simulink model "verify_THB_P_adapter_mdl"  (R2016b)
settings: Solver=ode45  StartTime=0  StopTime=600  MaxStep=10  RelTol=1e-3  EnableMultiTasking=on
libraries: carnot x2, simulink x1
settings Model: Creator=drhf  LastModifiedBy=drhf
settings DataIOCC: SaveFormat=Array  SignalLoggingSaveFormat=ModelDataLogs
settings OptimizationCC: ExpressionDepthLimit=2147483647  LifeSpan=inf
settings DebuggingCC: UnderspecifiedInitializationDetection=Classic  MergeDetectMultiDrivingBlocksExec=none  SolverPrmCheckMsg=warning  FcnCallInpInsideContextMsg=warning  StateNameClashWarn=warning  SFUnexpectedBacktrackingDiag=warning  SFNoUnconditionalDefaultTransitionDiag=warning  SFExecutionAtInitializationDiag=none
settings HardwareCC: ProdBitPerPointer=32  ProdBitPerSizeT=32  ProdBitPerPtrDiffT=32  ProdLargestAtomicFloat=None  ProdIntDivRoundTo=Undefined  ProdEndianess=Unspecified  ProdWordSize=32  ProdHWDeviceType=32-bit Generic
settings ModelReferenceCC: PropagateSignalLabelsOutOfModel=off
settings GRTTargetCC: TargetLangStandard=C89/C90 (ANSI)  GeneratePreprocessorConditionals=Disable all  CombineOutputUpdateFcns=off  GRTInterface=on
settings ConfigComp: CovMetricSettings=dw  CovHtmlReporting=on  CovSaveCumulativeToWorkspaceVar=on  CovSaveSingleToWorkspaceVar=on  CovExternalEMLEnable=off

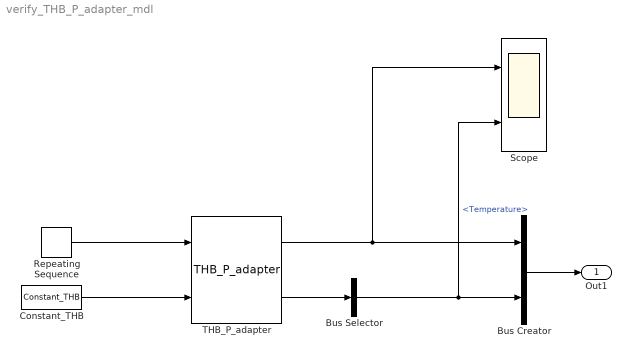
== system verify_THB_P_adapter_mdl ==
  Bus Creator : BusCreator  Inputs=2
  Bus Selector : BusSelector  OutputSignals=Temperature
  Constant_THB : carnot/Source/Simple/Constant_THB  t=40  mdot=600/3600  p=1e5  mID=No Pressure Drop  fluid=Water  mix=0  mix2=0  mix3=0  dia=0.02  hgt=0
  Repeating Sequence : simulink/Sources/Repeating Sequence  rep_seq_t=[0 100 200 400 500 600]  rep_seq_y=[20 20 30 30 10 10]
  Scope : Scope  NumInputPorts=2
  THB_P_adapter : carnot/Load/Houses/ventilation_heating/THB_P_adapter  mass=1  ua=800*5*5/0.2*0.022*3.1415  t0=20
  Out1 : Outport
  wires:
  THB_P_adapter/2 -> Bus Selector/1
  Constant_THB/1 -> THB_P_adapter/2
  Repeating Sequence/1 -> THB_P_adapter/1
  THB_P_adapter/1 -> Scope/1, Bus Creator/1
  Bus Selector/1 -> Scope/2, Bus Creator/2  "<Temperature>"
  Bus Creator/1 -> Out1/1
